simulink model "Simple_State_Observer"  (R2024b)
settings: Solver=VariableStepAuto  StartTime=0.0  StopTime=10.0  RelTol=1e-3
undefined symbols (not defined in the file or in its folder): degs2rpm, denHPF, numHPF
settings Model: Creator=llp  LastModifiedBy=llp

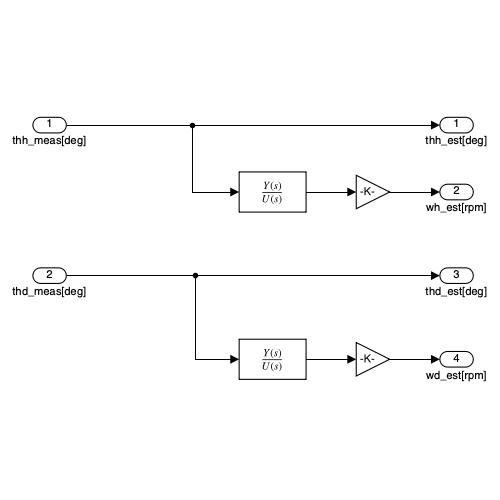
[thumbnail: Simulink's stored preview of the top-level diagram]
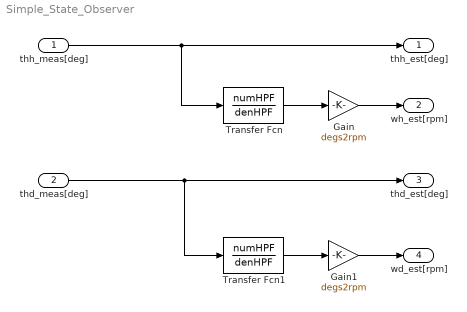
== system Simple_State_Observer ==
  thh_meas[deg] : Inport
  thd_meas[deg] : Inport  Port=2
  Gain : Gain  Gain=degs2rpm
  Gain1 : Gain  Gain=degs2rpm
  Transfer Fcn : TransferFcn  Numerator=numHPF  Denominator=denHPF
  Transfer Fcn1 : TransferFcn  Numerator=numHPF  Denominator=denHPF
  thh_est[deg] : Outport
  wh_est[rpm] : Outport  Port=2
  thd_est[deg] : Outport  Port=3
  wd_est[rpm] : Outport  Port=4
  wires:
  thh_meas[deg]/1 -> Transfer Fcn/1, thh_est[deg]/1
  Transfer Fcn/1 -> Gain/1
  Transfer Fcn1/1 -> Gain1/1
  thd_meas[deg]/1 -> Transfer Fcn1/1, thd_est[deg]/1
  Gain/1 -> wh_est[rpm]/1
  Gain1/1 -> wd_est[rpm]/1
